simulink model "QMUAV_Simulation_Model_V2"  (R2019b)
settings: Solver=VariableStepAuto  StartTime=0.0  StopTime=10.0  RelTol=1e-3
values from neighbouring files (symbols this model uses):
  Ix = 1    [QMUAV_Simulation_Model_Mscript.m]
  Iy = 1    [QMUAV_Simulation_Model_Mscript.m]
  Iz = 1    [QMUAV_Simulation_Model_Mscript.m]
  Kd_alt = 0    [QMUAV_Simulation_Model_Mscript.m]
  Kd_pitch = 0    [QMUAV_Simulation_Model_Mscript.m]
  Kd_roll = 0    [QMUAV_Simulation_Model_Mscript.m]
  Kd_x = 0    [QMUAV_Simulation_Model_Mscript.m]
  Kd_y = 0    [QMUAV_Simulation_Model_Mscript.m]
  Kd_yaw = 0    [QMUAV_Simulation_Model_Mscript.m]
  Ki_alt = 0    [QMUAV_Simulation_Model_Mscript.m]
  Ki_pitch = 0    [QMUAV_Simulation_Model_Mscript.m]
  Ki_roll = 0    [QMUAV_Simulation_Model_Mscript.m]
  Ki_x = 0    [QMUAV_Simulation_Model_Mscript.m]
  Ki_y = 0    [QMUAV_Simulation_Model_Mscript.m]
  Ki_yaw = 0    [QMUAV_Simulation_Model_Mscript.m]
  Kp_alt = 0    [QMUAV_Simulation_Model_Mscript.m]
  Kp_pitch = 0    [QMUAV_Simulation_Model_Mscript.m]
  Kp_roll = 0    [QMUAV_Simulation_Model_Mscript.m]
  Kp_x = 0    [QMUAV_Simulation_Model_Mscript.m]
  Kp_y = 0    [QMUAV_Simulation_Model_Mscript.m]
  Kp_yaw = 0    [QMUAV_Simulation_Model_Mscript.m]
  m = 1    [QMUAV_Simulation_Model_Mscript.m]
  maxPWM = 255    [QMUAV_Simulation_Model_Mscript.m]
  minPWM = 0    [QMUAV_Simulation_Model_Mscript.m]
  rx = 1    [QMUAV_Simulation_Model_Mscript.m]
  ry = 1    [QMUAV_Simulation_Model_Mscript.m]
  setpoint_alt = 0    [QMUAV_Simulation_Model_Mscript.m]
  setpoint_x = 0    [QMUAV_Simulation_Model_Mscript.m]
  setpoint_y = 0    [QMUAV_Simulation_Model_Mscript.m]
libraries: simulink x6
settings Model: Creator=alexc  LastModifiedBy=alexc

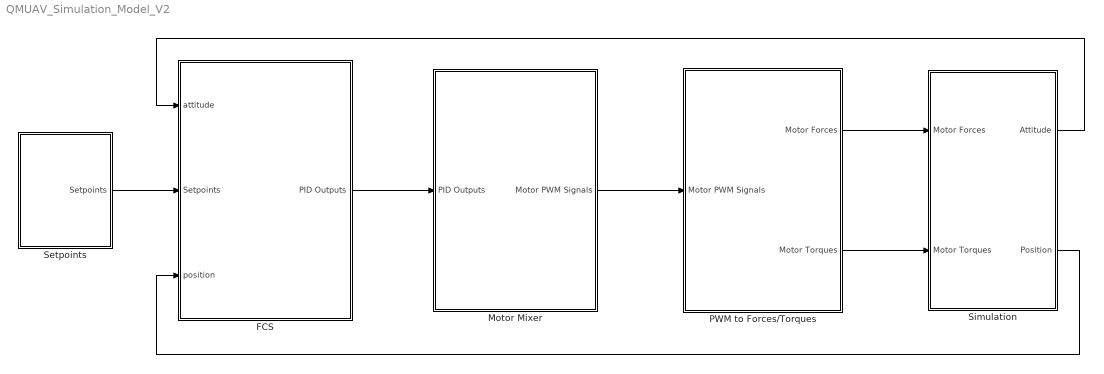
== system QMUAV_Simulation_Model_V2 ==
  FCS : Subsystem
  Motor Mixer : Subsystem
  PWM to Forces/Torques : Subsystem
  Setpoints : Subsystem
  Simulation : Subsystem
  wires:
  FCS/1(PID Outputs) -> Motor Mixer/1(PID Outputs)
  Motor Mixer/1(Motor PWM Signals) -> PWM to Forces/Torques/1(Motor PWM Signals)
  PWM to Forces/Torques/1(Motor Forces) -> Simulation/1(Motor Forces)
  Simulation/1(Attitude) -> FCS/1(attitude)
  Simulation/2(Position) -> FCS/3(position)
  Setpoints/1(Setpoints) -> FCS/2(Setpoints)
  PWM to Forces/Torques/2(Motor Torques) -> Simulation/2(Motor Torques)

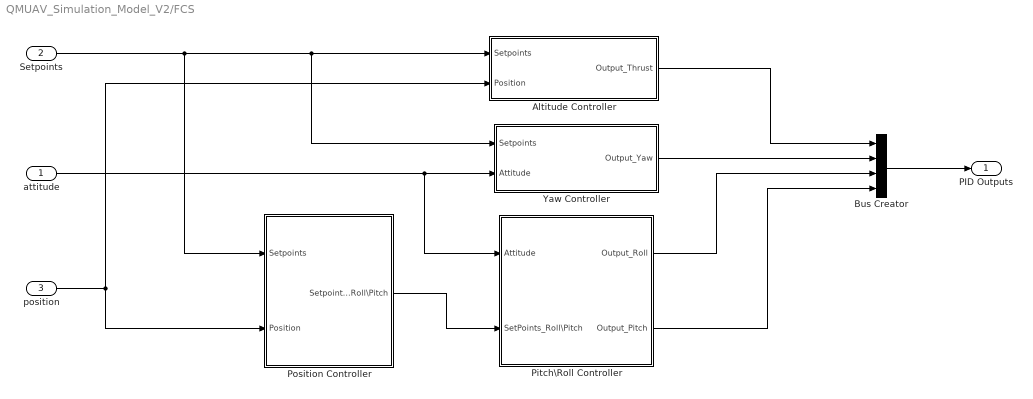
== system QMUAV_Simulation_Model_V2/FCS ==
  attitude : Inport
  Setpoints : Inport  Port=2
  position : Inport  Port=3
  Altitude Controller : Subsystem
  Bus Creator : BusCreator  Inputs=4
  Pitch\Roll Controller : Subsystem
  Position Controller : Subsystem
  Yaw Controller : Subsystem
  PID Outputs : Outport
  wires:
  Bus Creator/1 -> PID Outputs/1
  Altitude Controller/1(Output_Thrust) -> Bus Creator/1
  Pitch\Roll Controller/1(Output_Roll) -> Bus Creator/3
  Yaw Controller/1(Output_Yaw) -> Bus Creator/2
  position/1 -> Position Controller/2(Position), Altitude Controller/2(Position)
  attitude/1 -> Pitch\Roll Controller/1(Attitude), Yaw Controller/2(Attitude)
  Setpoints/1 -> Position Controller/1(Setpoints), Yaw Controller/1(Setpoints), Altitude Controller/1(Setpoints)
  Pitch\Roll Controller/2(Output_Pitch) -> Bus Creator/4
  Position Controller/1(Setpoints_Roll\Pitch) -> Pitch\Roll Controller/2(SetPoints_Roll\Pitch)

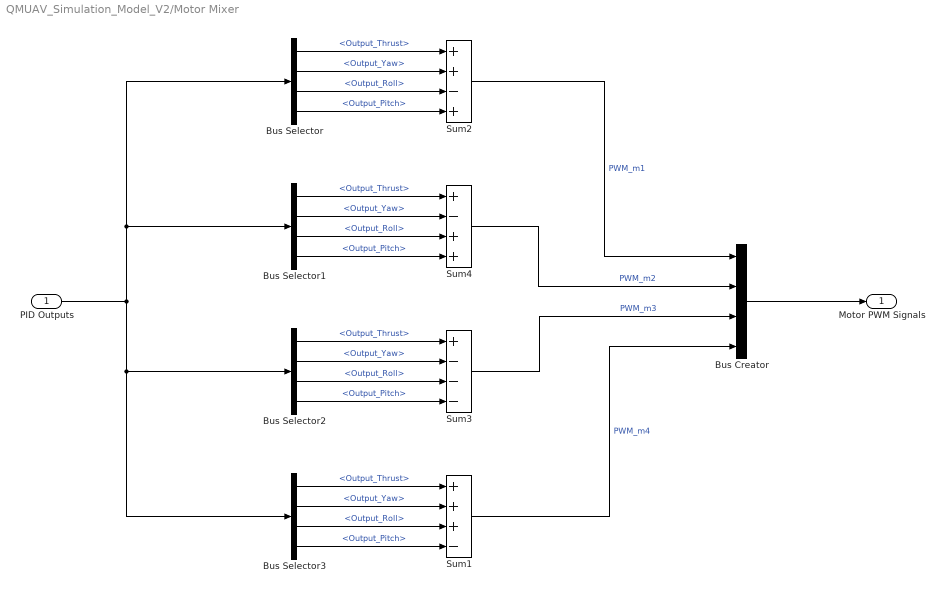
== system QMUAV_Simulation_Model_V2/Motor Mixer ==
  PID Outputs : Inport
  Bus Creator : BusCreator  Inputs=4
  Bus Selector{,1..3} (4 alike) : BusSelector  OutputSignals=Output_Thrust,Output_Yaw,Output_Roll,Output_Pitch
  Sum1 : Sum  Inputs=+++-
  Sum2 : Sum  Inputs=++-+
  Sum3 : Sum  Inputs=+---
  Sum4 : Sum  Inputs=+-++
  Motor PWM Signals : Outport
  wires:
  Sum4/1 -> Bus Creator/2  "PWM_m2"
  Sum3/1 -> Bus Creator/3  "PWM_m3"
  Sum1/1 -> Bus Creator/4  "PWM_m4"
  Sum2/1 -> Bus Creator/1  "PWM_m1"
  PID Outputs/1 -> Bus Selector3/1, Bus Selector2/1, Bus Selector1/1, Bus Selector/1
  Bus Selector/1 -> Sum2/1  "<Output_Thrust>"
  Bus Selector/2 -> Sum2/2  "<Output_Yaw>"
  Bus Selector/3 -> Sum2/3  "<Output_Roll>"
  Bus Selector/4 -> Sum2/4  "<Output_Pitch>"
  Bus Selector1/1 -> Sum4/1  "<Output_Thrust>"
  Bus Selector1/2 -> Sum4/2  "<Output_Yaw>"
  Bus Selector1/3 -> Sum4/3  "<Output_Roll>"
  Bus Selector1/4 -> Sum4/4  "<Output_Pitch>"
  Bus Selector2/1 -> Sum3/1  "<Output_Thrust>"
  Bus Selector2/2 -> Sum3/2  "<Output_Yaw>"
  Bus Selector2/3 -> Sum3/3  "<Output_Roll>"
  Bus Selector2/4 -> Sum3/4  "<Output_Pitch>"
  Bus Selector3/1 -> Sum1/1  "<Output_Thrust>"
  Bus Selector3/2 -> Sum1/2  "<Output_Yaw>"
  Bus Selector3/3 -> Sum1/3  "<Output_Roll>"
  Bus Selector3/4 -> Sum1/4  "<Output_Pitch>"
  Bus Creator/1 -> Motor PWM Signals/1

== system QMUAV_Simulation_Model_V2/PWM to Forces//Torques ==
  Motor PWM Signals : Inport
  Forces Lookup : Subsystem
  Torques Lookup : Subsystem
  Motor Forces : Outport
  Motor Torques : Outport  Port=2
  wires:
  Motor PWM Signals/1 -> Torques Lookup/1(In1), Forces Lookup/1(In1)
  Forces Lookup/1(Out1) -> Motor Forces/1
  Torques Lookup/1(Out1) -> Motor Torques/1

== system QMUAV_Simulation_Model_V2/Setpoints ==
  " " : Constant  Value=setpoint_alt
  Bus Creator : BusCreator  Inputs=4
  Constant1 : Constant  Value=setpoint_x
  Constant2 : Constant  Value=setpoint_y
  Constant3 : Constant  Value=setpoint_x
  Setpoints : Outport
  wires:
  Bus Creator/1 -> Setpoints/1
  " "/1 -> Bus Creator/1  "setpoint_alt"
  Constant1/1 -> Bus Creator/3  "setpoint_x"
  Constant2/1 -> Bus Creator/4  "setpoint_y"
  Constant3/1 -> Bus Creator/2  "setpoint_Yaw"

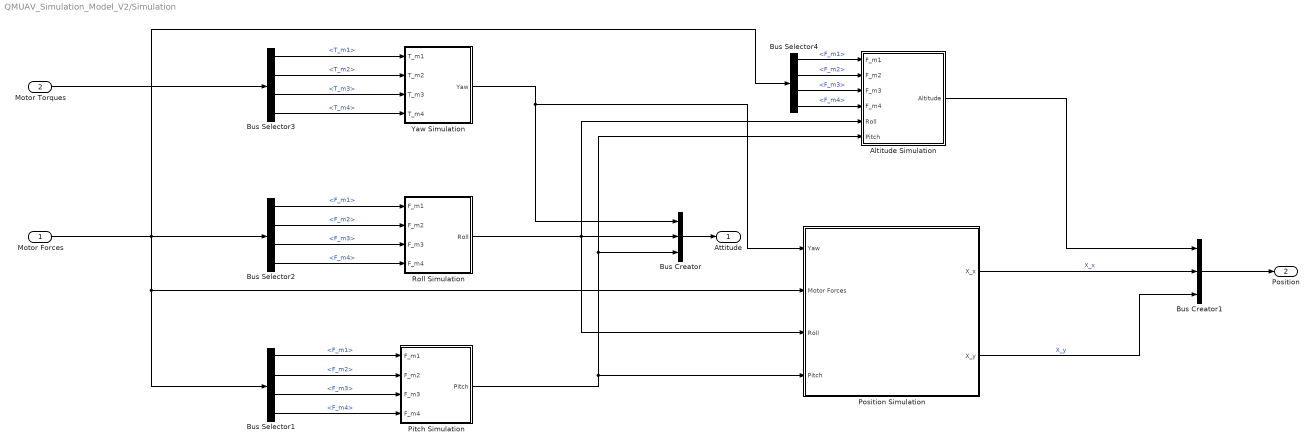
== system QMUAV_Simulation_Model_V2/Simulation ==
  Motor Forces : Inport
  Motor Torques : Inport  Port=2
  Altitude Simulation : Subsystem
  Bus Creator : BusCreator  Inputs=3
  Bus Creator1 : BusCreator  Inputs=3
  Bus Selector1 : BusSelector  OutputSignals=F_m1,F_m2,F_m3,F_m4
  Bus Selector2 : BusSelector  OutputSignals=F_m1,F_m2,F_m3,F_m4
  Bus Selector3 : BusSelector  OutputSignals=T_m1,T_m2,T_m3,T_m4
  Bus Selector4 : BusSelector  OutputSignals=F_m1,F_m2,F_m3,F_m4
  Pitch Simulation : Subsystem
  Position Simulation : Subsystem
  Roll Simulation : Subsystem
  Yaw Simulation : Subsystem
  Attitude : Outport
  Position : Outport  Port=2
  wires:
  Yaw Simulation/1(Yaw) -> Bus Creator/1, Position Simulation/1(Yaw)
  Roll Simulation/1(Roll) -> Position Simulation/3(Roll), Bus Creator/2, Altitude Simulation/5(Roll)
  Pitch Simulation/1(Pitch) -> Altitude Simulation/6(Pitch), Bus Creator/3, Position Simulation/4(Pitch)
  Motor Forces/1 -> Bus Selector1/1, Position Simulation/2(Motor Forces), Bus Selector2/1, Bus Selector4/1
  Bus Selector3/1 -> Yaw Simulation/1(T_m1)  "<T_m1>"
  Bus Selector3/2 -> Yaw Simulation/2(T_m2)  "<T_m2>"
  Bus Selector3/3 -> Yaw Simulation/3(T_m3)  "<T_m3>"
  Bus Selector3/4 -> Yaw Simulation/4(T_m4)  "<T_m4>"
  Bus Selector2/1 -> Roll Simulation/1(F_m1)  "<F_m1>"
  Bus Selector2/2 -> Roll Simulation/2(F_m2)  "<F_m2>"
  Bus Selector2/3 -> Roll Simulation/3(F_m3)  "<F_m3>"
  Bus Selector2/4 -> Roll Simulation/4(F_m4)  "<F_m4>"
  Bus Selector1/1 -> Pitch Simulation/1(F_m1)  "<F_m1>"
  Bus Selector1/2 -> Pitch Simulation/2(F_m2)  "<F_m2>"
  Bus Selector1/3 -> Pitch Simulation/3(F_m3)  "<F_m3>"
  Bus Selector1/4 -> Pitch Simulation/4(F_m4)  "<F_m4>"
  Bus Selector4/1 -> Altitude Simulation/1(F_m1)  "<F_m1>"
  Bus Selector4/2 -> Altitude Simulation/2(F_m2)  "<F_m2>"
  Bus Selector4/3 -> Altitude Simulation/3(F_m3)  "<F_m3>"
  Bus Selector4/4 -> Altitude Simulation/4(F_m4)  "<F_m4>"
  Bus Creator/1 -> Attitude/1
  Bus Creator1/1 -> Position/1
  Position Simulation/1(X_x) -> Bus Creator1/2  "X_x"
  Position Simulation/2(X_y) -> Bus Creator1/3  "X_y"
  Altitude Simulation/1(Altitude) -> Bus Creator1/1
  Motor Torques/1 -> Bus Selector3/1

== system QMUAV_Simulation_Model_V2/FCS/Altitude Controller ==
  Setpoints : Inport
  Position : Inport  Port=2
  Bus Selector : BusSelector  OutputSignals=Altitude
  Bus Selector1 : BusSelector  OutputSignals=setpoint_alt
  PID Controller : simulink/Continuous/PID Controller  Controller=PID  Form=Parallel  TimeDomain=Continuous-time  SampleTime=-1  IntegratorMethod=Forward Euler  FilterMethod=Forward Euler  ControllerParametersSource=internal  P=Kp_alt  I=Ki_alt  D=Kd_alt  UseFilter=on  N=100  TunerSelectOption=Transfer Function Based (PID Tuner App)  InitialConditionSource=internal  InitialConditionForIntegrator=0  InitialConditionForFilter=0  DifferentiatorICPrevScaledInput=0  ExternalReset=none  TrackingMode=off  Kt=1  LimitOutput=on  UpperSaturationLimit=maxPWM  LowerSaturationLimit=minPWM  LinearizeAsGain=on  AntiWindupMode=none  Kb=1  POutMin=[]  POutMax=[]  IOutMin=[]  IOutMax=[]  DOutMin=[]  DOutMax=[]  NOutMin=[]  NOutMax=[]  SumOutMin=[]  SumOutMax=[]  SaturationOutMin=[]  SaturationOutMax=[]  PParamMin=[]  PParamMax=[]  IParamMin=[]  IParamMax=[]  DParamMin=[]  DParamMax=[]  NParamMin=[]  NParamMax=[]  KbParamMin=[]  KbParamMax=[]  KtParamMin=[]  KtParamMax=[]  KbOutMin=[]  KbOutMax=[]  KtOutMin=[]  KtOutMax=[]  IntegratorOutMin=[]  IntegratorOutMax=[]  FilterOutMin=[]  FilterOutMax=[]  SumI1OutMin=[]  SumI1OutMax=[]  SumI2OutMin=[]  SumI2OutMax=[]  SumI3OutMin=[]  SumI3OutMax=[]  SumI4OutMin=[]  SumI4OutMax=[]  SumDOutMin=[]  SumDOutMax=[]  DifferentiatorOutMin=[]  DifferentiatorOutMax=[]  FilterDiffOutCoefMin=[]  FilterDiffOutCoefMax=[]  ReciprocalOutMin=[]  ReciprocalOutMax=[]  SumDenOutMin=[]  SumDenOutMax=[]  SumNumOutMin=[]  SumNumOutMax=[]  DivideOutMin=[]  DivideOutMax=[]  IntegratorContinuousStateAttributes=''  IntegratorStateMustResolveToSignalObject=off  IntegratorRTWStateStorageClass=Auto  FilterContinuousStateAttributes=''  FilterStateMustResolveToSignalObject=off  FilterRTWStateStorageClass=Auto  ParallelPVariant=InternalParameters  IdealPVariant=Disabled  IVariant=InternalParameters  DVariant=InternalParameters  IntegratorVariant=Continuous  SatVariant=Enabled  AWVariant=Passthrough  PCopyVariant=Disabled  TRVariant=Disabled  FdbkBlocksVariant=Forward  IdealPFdbkVariant=Disabled  SatFdbkVariant=Disabled  DerivativeFilterVariant=ContFilter  NVariant=InternalParameters  NCopyVariant=Disabled  FilterICVariant=InternalICsFilter  IntegratorICVariant=InternalICs  ExternalResetVariant=Disabled  TRSumVariant=Passthrough  SumFdbkVariant=Disabled  SumVariant=Sum_PID
  Sum : Sum  Inputs=|+-
  Output_Thrust : Outport
  wires:
  Bus Selector/1 -> Sum/1  "<Altitude>"
  Sum/1 -> PID Controller/1  "Error_Altitude"
  PID Controller/1 -> Output_Thrust/1  "Output_Thrust"
  Position/1 -> Bus Selector/1
  Setpoints/1 -> Bus Selector1/1
  Bus Selector1/1 -> Sum/2  "<setpoint_alt>"

== system QMUAV_Simulation_Model_V2/FCS/Pitch\Roll Controller ==
  Attitude : Inport
  SetPoints_Roll\Pitch : Inport  Port=2
  Pitch Controller : Subsystem
  Roll Controller : Subsystem
  Output_Roll : Outport
  Output_Pitch : Outport  Port=2
  wires:
  SetPoints_Roll\Pitch/1 -> Pitch Controller/1(Setpoints), Roll Controller/1(Setpoints)
  Attitude/1 -> Pitch Controller/2(Attitude), Roll Controller/2(Attitude)
  Roll Controller/1(Output_Roll) -> Output_Roll/1
  Pitch Controller/1(Output_Pitch) -> Output_Pitch/1

== system QMUAV_Simulation_Model_V2/FCS/Position Controller ==
  Setpoints : Inport
  Position : Inport  Port=2
  Bus Creator : BusCreator  Inputs=2
  X_x Controller : Subsystem
  X_y Controller : Subsystem
  Setpoints_Roll\Pitch : Outport
  wires:
  Position/1 -> X_y Controller/2(Position), X_x Controller/2(Position)
  Setpoints/1 -> X_y Controller/1(Setpoints), X_x Controller/1(Setpoints)
  X_x Controller/1(setpoint_pitch) -> Bus Creator/1
  X_y Controller/1(setpoint_roll) -> Bus Creator/2
  Bus Creator/1 -> Setpoints_Roll\Pitch/1

== system QMUAV_Simulation_Model_V2/FCS/Yaw Controller ==
  Setpoints : Inport
  Attitude : Inport  Port=2
  Bus Selector : BusSelector  OutputSignals=Yaw
  Bus Selector1 : BusSelector  OutputSignals=setpoint_Yaw
  PID Controller1 : simulink/Continuous/PID Controller  Controller=PID  Form=Parallel  TimeDomain=Continuous-time  SampleTime=-1  IntegratorMethod=Forward Euler  FilterMethod=Forward Euler  ControllerParametersSource=internal  P=Kp_yaw  I=Ki_yaw  D=Kd_yaw  UseFilter=on  N=100  TunerSelectOption=Transfer Function Based (PID Tuner App)  InitialConditionSource=internal  InitialConditionForIntegrator=0  InitialConditionForFilter=0  DifferentiatorICPrevScaledInput=0  ExternalReset=none  TrackingMode=off  Kt=1  LimitOutput=on  UpperSaturationLimit=maxPWM  LowerSaturationLimit=minPWM  LinearizeAsGain=on  AntiWindupMode=none  Kb=1  POutMin=[]  POutMax=[]  IOutMin=[]  IOutMax=[]  DOutMin=[]  DOutMax=[]  NOutMin=[]  NOutMax=[]  SumOutMin=[]  SumOutMax=[]  SaturationOutMin=[]  SaturationOutMax=[]  PParamMin=[]  PParamMax=[]  IParamMin=[]  IParamMax=[]  DParamMin=[]  DParamMax=[]  NParamMin=[]  NParamMax=[]  KbParamMin=[]  KbParamMax=[]  KtParamMin=[]  KtParamMax=[]  KbOutMin=[]  KbOutMax=[]  KtOutMin=[]  KtOutMax=[]  IntegratorOutMin=[]  IntegratorOutMax=[]  FilterOutMin=[]  FilterOutMax=[]  SumI1OutMin=[]  SumI1OutMax=[]  SumI2OutMin=[]  SumI2OutMax=[]  SumI3OutMin=[]  SumI3OutMax=[]  SumI4OutMin=[]  SumI4OutMax=[]  SumDOutMin=[]  SumDOutMax=[]  DifferentiatorOutMin=[]  DifferentiatorOutMax=[]  FilterDiffOutCoefMin=[]  FilterDiffOutCoefMax=[]  ReciprocalOutMin=[]  ReciprocalOutMax=[]  SumDenOutMin=[]  SumDenOutMax=[]  SumNumOutMin=[]  SumNumOutMax=[]  DivideOutMin=[]  DivideOutMax=[]  IntegratorContinuousStateAttributes=''  IntegratorStateMustResolveToSignalObject=off  IntegratorRTWStateStorageClass=Auto  FilterContinuousStateAttributes=''  FilterStateMustResolveToSignalObject=off  FilterRTWStateStorageClass=Auto  ParallelPVariant=InternalParameters  IdealPVariant=Disabled  IVariant=InternalParameters  DVariant=InternalParameters  IntegratorVariant=Continuous  SatVariant=Enabled  AWVariant=Passthrough  PCopyVariant=Disabled  TRVariant=Disabled  FdbkBlocksVariant=Forward  IdealPFdbkVariant=Disabled  SatFdbkVariant=Disabled  DerivativeFilterVariant=ContFilter  NVariant=InternalParameters  NCopyVariant=Disabled  FilterICVariant=InternalICsFilter  IntegratorICVariant=InternalICs  ExternalResetVariant=Disabled  TRSumVariant=Passthrough  SumFdbkVariant=Disabled  SumVariant=Sum_PID
  Sum1 : Sum  Inputs=|+-
  Output_Yaw : Outport
  wires:
  PID Controller1/1 -> Output_Yaw/1  "Output_Yaw"
  Sum1/1 -> PID Controller1/1  "Error_Yaw"
  Bus Selector/1 -> Sum1/1  "<Yaw>"
  Attitude/1 -> Bus Selector/1
  Setpoints/1 -> Bus Selector1/1
  Bus Selector1/1 -> Sum1/2  "<setpoint_Yaw>"

== system QMUAV_Simulation_Model_V2/PWM to Forces//Torques/Forces Lookup ==
  In1 : Inport
  1-D Lookup Table{,1..3} (4 alike) : Lookup_n-D  NumberOfTableDimensions=1  BreakpointsForDimension1=[-5:5]  Table=tanh([-5:5])  InternalRulePriority=Speed  RndMeth=Simplest  InputSameDT=on
  Bus Creator : BusCreator  Inputs=4
  Bus Selector : BusSelector  OutputSignals=PWM_m1,PWM_m2,PWM_m3,PWM_m4
  Out1 : Outport
  wires:
  Bus Selector/2 -> 1-D Lookup Table1/1  "<PWM_m2>"
  Bus Selector/1 -> 1-D Lookup Table/1  "<PWM_m1>"
  1-D Lookup Table/1 -> Bus Creator/1  "F_m1"
  1-D Lookup Table3/1 -> Bus Creator/4  "F_m4"
  1-D Lookup Table2/1 -> Bus Creator/3  "F_m3"
  Bus Selector/3 -> 1-D Lookup Table2/1  "<PWM_m3>"
  Bus Selector/4 -> 1-D Lookup Table3/1  "<PWM_m4>"
  1-D Lookup Table1/1 -> Bus Creator/2  "F_m2"
  In1/1 -> Bus Selector/1
  Bus Creator/1 -> Out1/1

== system QMUAV_Simulation_Model_V2/PWM to Forces//Torques/Torques Lookup ==
  In1 : Inport
  1-D Lookup Table{,1..3} (4 alike) : Lookup_n-D  NumberOfTableDimensions=1  BreakpointsForDimension1=[-5:5]  Table=tanh([-5:5])  InternalRulePriority=Speed  RndMeth=Simplest  InputSameDT=on
  Bus Creator : BusCreator  Inputs=4
  Bus Selector : BusSelector  OutputSignals=PWM_m1,PWM_m2,PWM_m3,PWM_m4
  Out1 : Outport
  wires:
  Bus Creator/1 -> Out1/1
  In1/1 -> Bus Selector/1
  1-D Lookup Table1/1 -> Bus Creator/2  "T_m2"
  Bus Selector/4 -> 1-D Lookup Table3/1  "<PWM_m4>"
  Bus Selector/3 -> 1-D Lookup Table2/1  "<PWM_m3>"
  1-D Lookup Table2/1 -> Bus Creator/3  "T_m3"
  1-D Lookup Table3/1 -> Bus Creator/4  "T_m4"
  1-D Lookup Table/1 -> Bus Creator/1  "T_m1"
  Bus Selector/1 -> 1-D Lookup Table/1  "<PWM_m1>"
  Bus Selector/2 -> 1-D Lookup Table1/1  "<PWM_m2>"

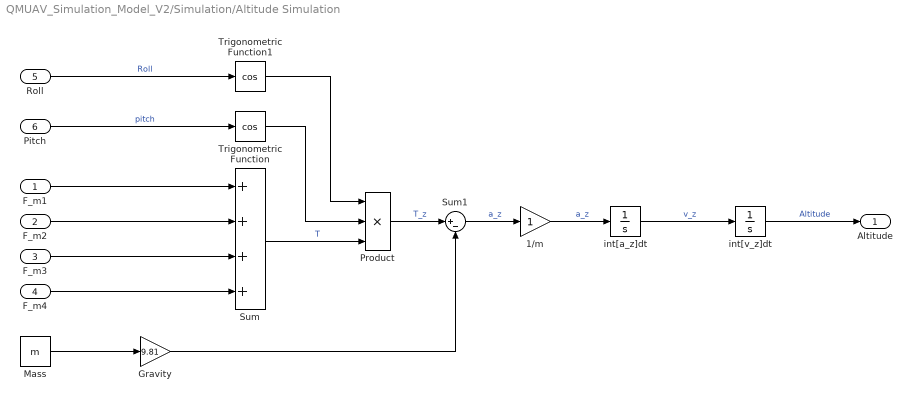
== system QMUAV_Simulation_Model_V2/Simulation/Altitude Simulation ==
  F_m1 : Inport
  F_m2 : Inport  Port=2
  F_m3 : Inport  Port=3
  F_m4 : Inport  Port=4
  Roll : Inport  Port=5
  Pitch : Inport  Port=6
  1/m : Gain
  Gravity : Gain  Gain=9.81
  Mass : Constant  Value=m
  Product : Product  Inputs=3
  Sum : Sum  Inputs=++++
  Sum1 : Sum  Inputs=|+-
  Trigonometric Function : Trigonometry  Operator=cos
  Trigonometric Function1 : Trigonometry  Operator=cos
  int[a_z]dt : Integrator
  int[v_z]dt : Integrator
  Altitude : Outport
  wires:
  1/m/1 -> int[a_z]dt/1  "a_z"
  F_m3/1 -> Sum/3
  F_m4/1 -> Sum/4
  F_m2/1 -> Sum/2
  int[a_z]dt/1 -> int[v_z]dt/1  "v_z"
  Sum/1 -> Product/3  "T"
  F_m1/1 -> Sum/1
  int[v_z]dt/1 -> Altitude/1  "Altitude"
  Sum1/1 -> 1/m/1  "a_z"
  Pitch/1 -> Trigonometric Function/1  "pitch"
  Roll/1 -> Trigonometric Function1/1  "Roll"
  Trigonometric Function/1 -> Product/2
  Trigonometric Function1/1 -> Product/1
  Product/1 -> Sum1/1  "T_z"
  Gravity/1 -> Sum1/2
  Mass/1 -> Gravity/1

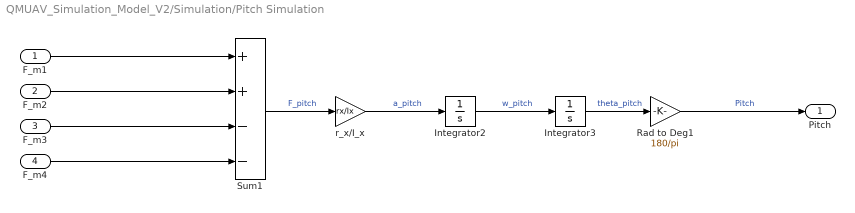
== system QMUAV_Simulation_Model_V2/Simulation/Pitch Simulation ==
  F_m1 : Inport
  F_m2 : Inport  Port=2
  F_m3 : Inport  Port=3
  F_m4 : Inport  Port=4
  Integrator2 : Integrator
  Integrator3 : Integrator
  Rad to Deg1 : Gain  Gain=180/pi
  Sum1 : Sum  Inputs=++--
  r_x/I_x : Gain  Gain=rx/Ix
  Pitch : Outport
  wires:
  F_m1/1 -> Sum1/1
  F_m2/1 -> Sum1/2
  Rad to Deg1/1 -> Pitch/1  "Pitch"
  r_x/I_x/1 -> Integrator2/1  "a_pitch"
  F_m4/1 -> Sum1/4
  F_m3/1 -> Sum1/3
  Integrator3/1 -> Rad to Deg1/1  "theta_pitch"
  Sum1/1 -> r_x/I_x/1  "F_pitch"
  Integrator2/1 -> Integrator3/1  "w_pitch"

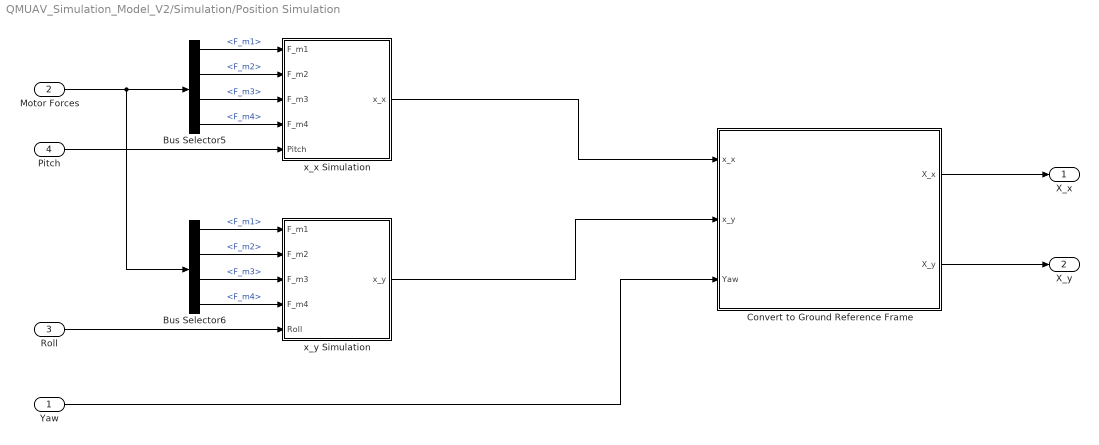
== system QMUAV_Simulation_Model_V2/Simulation/Position Simulation ==
  Yaw : Inport
  Motor Forces : Inport  Port=2
  Roll : Inport  Port=3
  Pitch : Inport  Port=4
  Bus Selector5 : BusSelector  OutputSignals=F_m1,F_m2,F_m3,F_m4
  Bus Selector6 : BusSelector  OutputSignals=F_m1,F_m2,F_m3,F_m4
  Convert to Ground Reference Frame : Subsystem
  x_x Simulation : Subsystem
  x_y Simulation : Subsystem
  X_x : Outport
  X_y : Outport  Port=2
  wires:
  Bus Selector6/4 -> x_y Simulation/4(F_m4)  "<F_m4>"
  Motor Forces/1 -> Bus Selector6/1, Bus Selector5/1
  Bus Selector5/2 -> x_x Simulation/2(F_m2)  "<F_m2>"
  Bus Selector5/1 -> x_x Simulation/1(F_m1)  "<F_m1>"
  Bus Selector6/3 -> x_y Simulation/3(F_m3)  "<F_m3>"
  Bus Selector6/2 -> x_y Simulation/2(F_m2)  "<F_m2>"
  x_y Simulation/1(x_y) -> Convert to Ground Reference Frame/2(x_y)
  x_x Simulation/1(x_x) -> Convert to Ground Reference Frame/1(x_x)
  Pitch/1 -> x_x Simulation/5(Pitch)
  Bus Selector6/1 -> x_y Simulation/1(F_m1)  "<F_m1>"
  Bus Selector5/3 -> x_x Simulation/3(F_m3)  "<F_m3>"
  Roll/1 -> x_y Simulation/5(Roll)
  Bus Selector5/4 -> x_x Simulation/4(F_m4)  "<F_m4>"
  Yaw/1 -> Convert to Ground Reference Frame/3(Yaw)
  Convert to Ground Reference Frame/1(X_x) -> X_x/1
  Convert to Ground Reference Frame/2(X_y) -> X_y/1

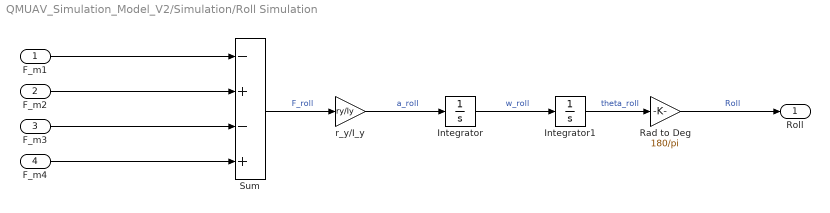
== system QMUAV_Simulation_Model_V2/Simulation/Roll Simulation ==
  F_m1 : Inport
  F_m2 : Inport  Port=2
  F_m3 : Inport  Port=3
  F_m4 : Inport  Port=4
  Integrator : Integrator
  Integrator1 : Integrator
  Rad to Deg : Gain  Gain=180/pi
  Sum : Sum  Inputs=-+-+
  r_y/I_y : Gain  Gain=ry/Iy
  Roll : Outport
  wires:
  F_m4/1 -> Sum/4
  F_m3/1 -> Sum/3
  Integrator/1 -> Integrator1/1  "w_roll"
  Sum/1 -> r_y/I_y/1  "F_roll"
  r_y/I_y/1 -> Integrator/1  "a_roll"
  F_m2/1 -> Sum/2
  Rad to Deg/1 -> Roll/1  "Roll"
  F_m1/1 -> Sum/1
  Integrator1/1 -> Rad to Deg/1  "theta_roll"

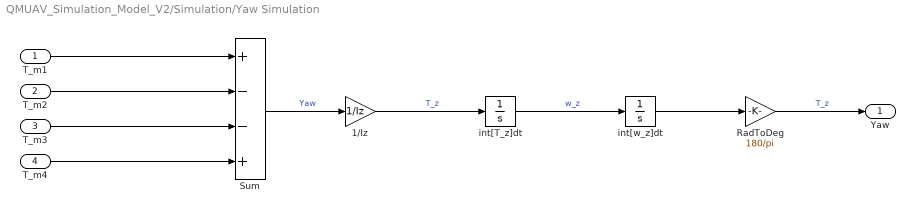
== system QMUAV_Simulation_Model_V2/Simulation/Yaw Simulation ==
  T_m1 : Inport
  T_m2 : Inport  Port=2
  T_m3 : Inport  Port=3
  T_m4 : Inport  Port=4
  1/Iz : Gain  Gain=1/Iz
  RadToDeg : Gain  Gain=180/pi
  Sum : Sum  Inputs=+--+
  int[T_z]dt : Integrator
  int[w_z]dt : Integrator
  Yaw : Outport
  wires:
  T_m4/1 -> Sum/4
  T_m3/1 -> Sum/3
  T_m2/1 -> Sum/2
  Sum/1 -> 1/Iz/1  "Yaw"
  T_m1/1 -> Sum/1
  1/Iz/1 -> int[T_z]dt/1  "T_z"
  int[T_z]dt/1 -> int[w_z]dt/1  "w_z"
  int[w_z]dt/1 -> RadToDeg/1
  RadToDeg/1 -> Yaw/1  "T_z"

== system QMUAV_Simulation_Model_V2/FCS/Pitch\Roll Controller/Pitch Controller ==
  Setpoints : Inport
  Attitude : Inport  Port=2
  Bus Selector : BusSelector  OutputSignals=Pitch
  Bus Selector1 : BusSelector  OutputSignals=setpoint_pitch
  PID Controller : simulink/Continuous/PID Controller  Controller=PID  Form=Parallel  TimeDomain=Continuous-time  SampleTime=-1  IntegratorMethod=Forward Euler  FilterMethod=Forward Euler  ControllerParametersSource=internal  P=Kp_pitch  I=Ki_pitch  D=Kd_pitch  UseFilter=on  N=100  TunerSelectOption=Transfer Function Based (PID Tuner App)  InitialConditionSource=internal  InitialConditionForIntegrator=0  InitialConditionForFilter=0  DifferentiatorICPrevScaledInput=0  ExternalReset=none  TrackingMode=off  Kt=1  LimitOutput=on  UpperSaturationLimit=maxPWM  LowerSaturationLimit=minPWM  LinearizeAsGain=on  AntiWindupMode=none  Kb=1  POutMin=[]  POutMax=[]  IOutMin=[]  IOutMax=[]  DOutMin=[]  DOutMax=[]  NOutMin=[]  NOutMax=[]  SumOutMin=[]  SumOutMax=[]  SaturationOutMin=[]  SaturationOutMax=[]  PParamMin=[]  PParamMax=[]  IParamMin=[]  IParamMax=[]  DParamMin=[]  DParamMax=[]  NParamMin=[]  NParamMax=[]  KbParamMin=[]  KbParamMax=[]  KtParamMin=[]  KtParamMax=[]  KbOutMin=[]  KbOutMax=[]  KtOutMin=[]  KtOutMax=[]  IntegratorOutMin=[]  IntegratorOutMax=[]  FilterOutMin=[]  FilterOutMax=[]  SumI1OutMin=[]  SumI1OutMax=[]  SumI2OutMin=[]  SumI2OutMax=[]  SumI3OutMin=[]  SumI3OutMax=[]  SumI4OutMin=[]  SumI4OutMax=[]  SumDOutMin=[]  SumDOutMax=[]  DifferentiatorOutMin=[]  DifferentiatorOutMax=[]  FilterDiffOutCoefMin=[]  FilterDiffOutCoefMax=[]  ReciprocalOutMin=[]  ReciprocalOutMax=[]  SumDenOutMin=[]  SumDenOutMax=[]  SumNumOutMin=[]  SumNumOutMax=[]  DivideOutMin=[]  DivideOutMax=[]  IntegratorContinuousStateAttributes=''  IntegratorStateMustResolveToSignalObject=off  IntegratorRTWStateStorageClass=Auto  FilterContinuousStateAttributes=''  FilterStateMustResolveToSignalObject=off  FilterRTWStateStorageClass=Auto  ParallelPVariant=InternalParameters  IdealPVariant=Disabled  IVariant=InternalParameters  DVariant=InternalParameters  IntegratorVariant=Continuous  SatVariant=Enabled  AWVariant=Passthrough  PCopyVariant=Disabled  TRVariant=Disabled  FdbkBlocksVariant=Forward  IdealPFdbkVariant=Disabled  SatFdbkVariant=Disabled  DerivativeFilterVariant=ContFilter  NVariant=InternalParameters  NCopyVariant=Disabled  FilterICVariant=InternalICsFilter  IntegratorICVariant=InternalICs  ExternalResetVariant=Disabled  TRSumVariant=Passthrough  SumFdbkVariant=Disabled  SumVariant=Sum_PID
  Sum : Sum  Inputs=|+-
  Output_Pitch : Outport
  wires:
  Attitude/1 -> Bus Selector/1
  Bus Selector/1 -> Sum/1  "<Pitch>"
  Bus Selector1/1 -> Sum/2  "<setpoint_pitch>"
  Setpoints/1 -> Bus Selector1/1
  PID Controller/1 -> Output_Pitch/1  "Output_Pitch"
  Sum/1 -> PID Controller/1  "Error_Pitch"

== system QMUAV_Simulation_Model_V2/FCS/Pitch\Roll Controller/Roll Controller ==
  Setpoints : Inport
  Attitude : Inport  Port=2
  Bus Selector : BusSelector  OutputSignals=Roll
  Bus Selector1 : BusSelector  OutputSignals=setpoint_roll
  PID Controller : simulink/Continuous/PID Controller  Controller=PID  Form=Parallel  TimeDomain=Continuous-time  SampleTime=-1  IntegratorMethod=Forward Euler  FilterMethod=Forward Euler  ControllerParametersSource=internal  P=Kp_roll  I=Ki_roll  D=Kd_roll  UseFilter=on  N=100  TunerSelectOption=Transfer Function Based (PID Tuner App)  InitialConditionSource=internal  InitialConditionForIntegrator=0  InitialConditionForFilter=0  DifferentiatorICPrevScaledInput=0  ExternalReset=none  TrackingMode=off  Kt=1  LimitOutput=on  UpperSaturationLimit=maxPWM  LowerSaturationLimit=minPWM  LinearizeAsGain=on  AntiWindupMode=none  Kb=1  POutMin=[]  POutMax=[]  IOutMin=[]  IOutMax=[]  DOutMin=[]  DOutMax=[]  NOutMin=[]  NOutMax=[]  SumOutMin=[]  SumOutMax=[]  SaturationOutMin=[]  SaturationOutMax=[]  PParamMin=[]  PParamMax=[]  IParamMin=[]  IParamMax=[]  DParamMin=[]  DParamMax=[]  NParamMin=[]  NParamMax=[]  KbParamMin=[]  KbParamMax=[]  KtParamMin=[]  KtParamMax=[]  KbOutMin=[]  KbOutMax=[]  KtOutMin=[]  KtOutMax=[]  IntegratorOutMin=[]  IntegratorOutMax=[]  FilterOutMin=[]  FilterOutMax=[]  SumI1OutMin=[]  SumI1OutMax=[]  SumI2OutMin=[]  SumI2OutMax=[]  SumI3OutMin=[]  SumI3OutMax=[]  SumI4OutMin=[]  SumI4OutMax=[]  SumDOutMin=[]  SumDOutMax=[]  DifferentiatorOutMin=[]  DifferentiatorOutMax=[]  FilterDiffOutCoefMin=[]  FilterDiffOutCoefMax=[]  ReciprocalOutMin=[]  ReciprocalOutMax=[]  SumDenOutMin=[]  SumDenOutMax=[]  SumNumOutMin=[]  SumNumOutMax=[]  DivideOutMin=[]  DivideOutMax=[]  IntegratorContinuousStateAttributes=''  IntegratorStateMustResolveToSignalObject=off  IntegratorRTWStateStorageClass=Auto  FilterContinuousStateAttributes=''  FilterStateMustResolveToSignalObject=off  FilterRTWStateStorageClass=Auto  ParallelPVariant=InternalParameters  IdealPVariant=Disabled  IVariant=InternalParameters  DVariant=InternalParameters  IntegratorVariant=Continuous  SatVariant=Enabled  AWVariant=Passthrough  PCopyVariant=Disabled  TRVariant=Disabled  FdbkBlocksVariant=Forward  IdealPFdbkVariant=Disabled  SatFdbkVariant=Disabled  DerivativeFilterVariant=ContFilter  NVariant=InternalParameters  NCopyVariant=Disabled  FilterICVariant=InternalICsFilter  IntegratorICVariant=InternalICs  ExternalResetVariant=Disabled  TRSumVariant=Passthrough  SumFdbkVariant=Disabled  SumVariant=Sum_PID
  Sum : Sum  Inputs=|+-
  Output_Roll : Outport
  wires:
  Attitude/1 -> Bus Selector/1
  Bus Selector/1 -> Sum/1  "<Roll>"
  Bus Selector1/1 -> Sum/2  "<setpoint_roll>"
  Setpoints/1 -> Bus Selector1/1
  PID Controller/1 -> Output_Roll/1  "Output_Roll"
  Sum/1 -> PID Controller/1  "Error_Roll"

== system QMUAV_Simulation_Model_V2/FCS/Position Controller/X_x Controller ==
  Setpoints : Inport
  Position : Inport  Port=2
  Bus Selector : BusSelector  OutputSignals=X_x
  Bus Selector1 : BusSelector  OutputSignals=setpoint_x
  PID Controller : simulink/Continuous/PID Controller  Controller=PID  Form=Parallel  TimeDomain=Continuous-time  SampleTime=-1  IntegratorMethod=Forward Euler  FilterMethod=Forward Euler  ControllerParametersSource=internal  P=Kp_x  I=Ki_x  D=Kd_x  UseFilter=on  N=100  TunerSelectOption=Transfer Function Based (PID Tuner App)  InitialConditionSource=internal  InitialConditionForIntegrator=0  InitialConditionForFilter=0  DifferentiatorICPrevScaledInput=0  ExternalReset=none  TrackingMode=off  Kt=1  LimitOutput=on  UpperSaturationLimit=maxPWM  LowerSaturationLimit=minPWM  LinearizeAsGain=on  AntiWindupMode=none  Kb=1  POutMin=[]  POutMax=[]  IOutMin=[]  IOutMax=[]  DOutMin=[]  DOutMax=[]  NOutMin=[]  NOutMax=[]  SumOutMin=[]  SumOutMax=[]  SaturationOutMin=[]  SaturationOutMax=[]  PParamMin=[]  PParamMax=[]  IParamMin=[]  IParamMax=[]  DParamMin=[]  DParamMax=[]  NParamMin=[]  NParamMax=[]  KbParamMin=[]  KbParamMax=[]  KtParamMin=[]  KtParamMax=[]  KbOutMin=[]  KbOutMax=[]  KtOutMin=[]  KtOutMax=[]  IntegratorOutMin=[]  IntegratorOutMax=[]  FilterOutMin=[]  FilterOutMax=[]  SumI1OutMin=[]  SumI1OutMax=[]  SumI2OutMin=[]  SumI2OutMax=[]  SumI3OutMin=[]  SumI3OutMax=[]  SumI4OutMin=[]  SumI4OutMax=[]  SumDOutMin=[]  SumDOutMax=[]  DifferentiatorOutMin=[]  DifferentiatorOutMax=[]  FilterDiffOutCoefMin=[]  FilterDiffOutCoefMax=[]  ReciprocalOutMin=[]  ReciprocalOutMax=[]  SumDenOutMin=[]  SumDenOutMax=[]  SumNumOutMin=[]  SumNumOutMax=[]  DivideOutMin=[]  DivideOutMax=[]  IntegratorContinuousStateAttributes=''  IntegratorStateMustResolveToSignalObject=off  IntegratorRTWStateStorageClass=Auto  FilterContinuousStateAttributes=''  FilterStateMustResolveToSignalObject=off  FilterRTWStateStorageClass=Auto  ParallelPVariant=InternalParameters  IdealPVariant=Disabled  IVariant=InternalParameters  DVariant=InternalParameters  IntegratorVariant=Continuous  SatVariant=Enabled  AWVariant=Passthrough  PCopyVariant=Disabled  TRVariant=Disabled  FdbkBlocksVariant=Forward  IdealPFdbkVariant=Disabled  SatFdbkVariant=Disabled  DerivativeFilterVariant=ContFilter  NVariant=InternalParameters  NCopyVariant=Disabled  FilterICVariant=InternalICsFilter  IntegratorICVariant=InternalICs  ExternalResetVariant=Disabled  TRSumVariant=Passthrough  SumFdbkVariant=Disabled  SumVariant=Sum_PID
  Sum : Sum  Inputs=|+-
  setpoint_pitch : Outport
  wires:
  Bus Selector1/1 -> Sum/2  "<setpoint_x>"
  Setpoints/1 -> Bus Selector1/1
  Sum/1 -> PID Controller/1  "Error_X_x"
  PID Controller/1 -> setpoint_pitch/1  "setpoint_pitch"
  Position/1 -> Bus Selector/1
  Bus Selector/1 -> Sum/1  "<X_x>"

== system QMUAV_Simulation_Model_V2/FCS/Position Controller/X_y Controller ==
  Setpoints : Inport
  Position : Inport  Port=2
  Bus Selector : BusSelector  OutputSignals=X_y
  Bus Selector1 : BusSelector  OutputSignals=setpoint_y
  PID Controller : simulink/Continuous/PID Controller  Controller=PID  Form=Parallel  TimeDomain=Continuous-time  SampleTime=-1  IntegratorMethod=Forward Euler  FilterMethod=Forward Euler  ControllerParametersSource=internal  P=Kp_y  I=Ki_y  D=Kd_y  UseFilter=on  N=100  TunerSelectOption=Transfer Function Based (PID Tuner App)  InitialConditionSource=internal  InitialConditionForIntegrator=0  InitialConditionForFilter=0  DifferentiatorICPrevScaledInput=0  ExternalReset=none  TrackingMode=off  Kt=1  LimitOutput=on  UpperSaturationLimit=maxPWM  LowerSaturationLimit=minPWM  LinearizeAsGain=on  AntiWindupMode=none  Kb=1  POutMin=[]  POutMax=[]  IOutMin=[]  IOutMax=[]  DOutMin=[]  DOutMax=[]  NOutMin=[]  NOutMax=[]  SumOutMin=[]  SumOutMax=[]  SaturationOutMin=[]  SaturationOutMax=[]  PParamMin=[]  PParamMax=[]  IParamMin=[]  IParamMax=[]  DParamMin=[]  DParamMax=[]  NParamMin=[]  NParamMax=[]  KbParamMin=[]  KbParamMax=[]  KtParamMin=[]  KtParamMax=[]  KbOutMin=[]  KbOutMax=[]  KtOutMin=[]  KtOutMax=[]  IntegratorOutMin=[]  IntegratorOutMax=[]  FilterOutMin=[]  FilterOutMax=[]  SumI1OutMin=[]  SumI1OutMax=[]  SumI2OutMin=[]  SumI2OutMax=[]  SumI3OutMin=[]  SumI3OutMax=[]  SumI4OutMin=[]  SumI4OutMax=[]  SumDOutMin=[]  SumDOutMax=[]  DifferentiatorOutMin=[]  DifferentiatorOutMax=[]  FilterDiffOutCoefMin=[]  FilterDiffOutCoefMax=[]  ReciprocalOutMin=[]  ReciprocalOutMax=[]  SumDenOutMin=[]  SumDenOutMax=[]  SumNumOutMin=[]  SumNumOutMax=[]  DivideOutMin=[]  DivideOutMax=[]  IntegratorContinuousStateAttributes=''  IntegratorStateMustResolveToSignalObject=off  IntegratorRTWStateStorageClass=Auto  FilterContinuousStateAttributes=''  FilterStateMustResolveToSignalObject=off  FilterRTWStateStorageClass=Auto  ParallelPVariant=InternalParameters  IdealPVariant=Disabled  IVariant=InternalParameters  DVariant=InternalParameters  IntegratorVariant=Continuous  SatVariant=Enabled  AWVariant=Passthrough  PCopyVariant=Disabled  TRVariant=Disabled  FdbkBlocksVariant=Forward  IdealPFdbkVariant=Disabled  SatFdbkVariant=Disabled  DerivativeFilterVariant=ContFilter  NVariant=InternalParameters  NCopyVariant=Disabled  FilterICVariant=InternalICsFilter  IntegratorICVariant=InternalICs  ExternalResetVariant=Disabled  TRSumVariant=Passthrough  SumFdbkVariant=Disabled  SumVariant=Sum_PID
  Sum : Sum  Inputs=|+-
  setpoint_roll : Outport
  wires:
  Bus Selector1/1 -> Sum/2  "<setpoint_y>"
  Setpoints/1 -> Bus Selector1/1
  Sum/1 -> PID Controller/1  "Error_X_y"
  PID Controller/1 -> setpoint_roll/1  "setpoint_roll"
  Position/1 -> Bus Selector/1
  Bus Selector/1 -> Sum/1  "<X_y>"

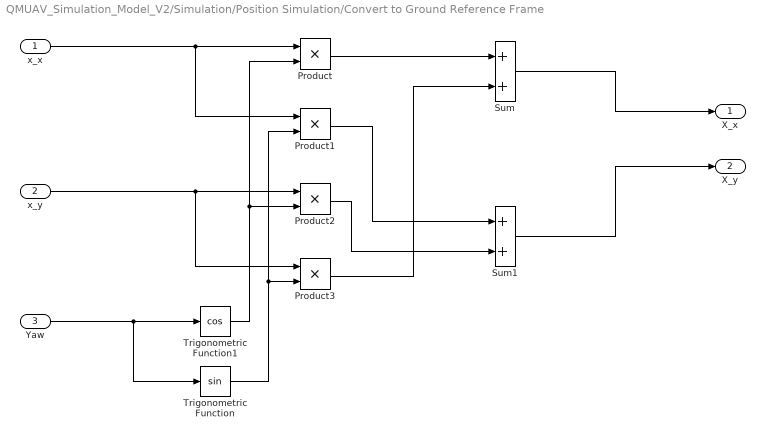
== system QMUAV_Simulation_Model_V2/Simulation/Position Simulation/Convert to Ground Reference Frame ==
  x_x : Inport
  x_y : Inport  Port=2
  Yaw : Inport  Port=3
  Product{,1..3} (4 alike) : Product
  Sum : Sum
  Sum1 : Sum
  Trigonometric Function : Trigonometry
  Trigonometric Function1 : Trigonometry  Operator=cos
  X_x : Outport
  X_y : Outport  Port=2
  wires:
  Yaw/1 -> Trigonometric Function1/1, Trigonometric Function/1
  Trigonometric Function1/1 -> Product2/2, Product/2
  x_x/1 -> Product1/1, Product/1
  Trigonometric Function/1 -> Product3/2, Product1/2
  x_y/1 -> Product3/1, Product2/1
  Product/1 -> Sum/1
  Product3/1 -> Sum/2
  Product1/1 -> Sum1/1
  Product2/1 -> Sum1/2
  Sum1/1 -> X_y/1
  Sum/1 -> X_x/1

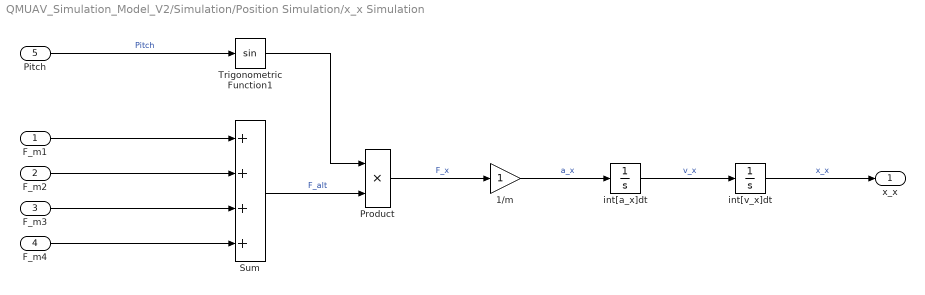
== system QMUAV_Simulation_Model_V2/Simulation/Position Simulation/x_x Simulation ==
  F_m1 : Inport
  F_m2 : Inport  Port=2
  F_m3 : Inport  Port=3
  F_m4 : Inport  Port=4
  Pitch : Inport  Port=5
  1/m : Gain
  Product : Product
  Sum : Sum  Inputs=++++
  Trigonometric Function1 : Trigonometry
  int[a_x]dt : Integrator
  int[v_x]dt : Integrator
  x_x : Outport
  wires:
  1/m/1 -> int[a_x]dt/1  "a_x"
  F_m3/1 -> Sum/3
  F_m4/1 -> Sum/4
  F_m2/1 -> Sum/2
  int[a_x]dt/1 -> int[v_x]dt/1  "v_x"
  Sum/1 -> Product/2  "F_alt"
  F_m1/1 -> Sum/1
  int[v_x]dt/1 -> x_x/1  "x_x"
  Pitch/1 -> Trigonometric Function1/1  "Pitch"
  Trigonometric Function1/1 -> Product/1
  Product/1 -> 1/m/1  "F_x"

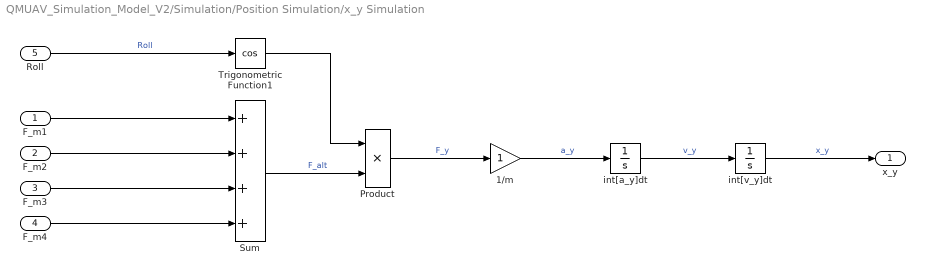
== system QMUAV_Simulation_Model_V2/Simulation/Position Simulation/x_y Simulation ==
  F_m1 : Inport
  F_m2 : Inport  Port=2
  F_m3 : Inport  Port=3
  F_m4 : Inport  Port=4
  Roll : Inport  Port=5
  1/m : Gain
  Product : Product
  Sum : Sum  Inputs=++++
  Trigonometric Function1 : Trigonometry  Operator=cos
  int[a_y]dt : Integrator
  int[v_y]dt : Integrator
  x_y : Outport
  wires:
  1/m/1 -> int[a_y]dt/1  "a_y"
  F_m3/1 -> Sum/3
  F_m4/1 -> Sum/4
  F_m2/1 -> Sum/2
  int[a_y]dt/1 -> int[v_y]dt/1  "v_y"
  Sum/1 -> Product/2  "F_alt"
  F_m1/1 -> Sum/1
  int[v_y]dt/1 -> x_y/1  "x_y"
  Roll/1 -> Trigonometric Function1/1  "Roll"
  Trigonometric Function1/1 -> Product/1
  Product/1 -> 1/m/1  "F_y"
